simulink model "exm070102"  (R2018a)
settings: Solver=ode45  StartTime=0.0  StopTime=10  MaxStep=0.01  RelTol=1e-3  EnableMultiTasking=on
settings Model: Creator=acer  LastModifiedBy=zyzhang
settings DataIOCC: LimitDataPoints=on  SaveFormat=Array  SignalLoggingSaveFormat=ModelDataLogs
settings OptimizationCC: ExpressionDepthLimit=2147483647  LifeSpan=inf
settings DebuggingCC: UnderspecifiedInitializationDetection=Classic  MergeDetectMultiDrivingBlocksExec=none  SolverPrmCheckMsg=warning  FcnCallInpInsideContextMsg=warning  StateNameClashWarn=warning  SFUnexpectedBacktrackingDiag=warning  SFNoUnconditionalDefaultTransitionDiag=warning  SFExecutionAtInitializationDiag=none
settings HardwareCC: ProdBitPerPointer=32  ProdBitPerSizeT=32  ProdBitPerPtrDiffT=32  ProdLargestAtomicFloat=None  ProdIntDivRoundTo=Undefined  ProdEndianess=Unspecified  ProdWordSize=32  ProdHWDeviceType=32-bit Generic
settings ModelReferenceCC: PropagateSignalLabelsOutOfModel=off
settings CodeAppCC: StateflowObjectComments=on
settings GRTTargetCC: TargetLangStandard=C89/C90 (ANSI)  GeneratePreprocessorConditionals=Disable all  CombineOutputUpdateFcns=off  GRTInterface=on
settings ConfigComp: CovMetricSettings=dw  CovHtmlReporting=on  CovSaveCumulativeToWorkspaceVar=on  CovSaveSingleToWorkspaceVar=on  CovExternalEMLEnable=off  CovSFcnEnable=off

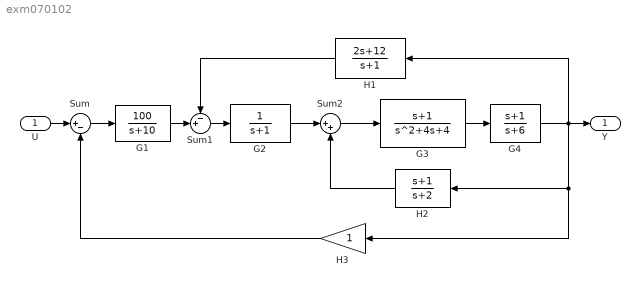
== system exm070102 ==
  U : Inport
  G1 : TransferFcn  Numerator=[100]  Denominator=[1 10]
  G2 : TransferFcn  Denominator=[1 1]
  G3 : TransferFcn  Numerator=[1 1]  Denominator=[1 4 4]
  G4 : TransferFcn  Numerator=[1 1]  Denominator=[1 6]
  H1 : TransferFcn  Numerator=[2 12]  Denominator=[1 1]
  H2 : TransferFcn  Numerator=[1 1]  Denominator=[1 2]
  H3 : Gain
  Sum : Sum  Inputs=|+-
  Sum1 : Sum  Inputs=-+|
  Sum2 : Sum  Inputs=|++
  Y : Outport
  wires:
  U/1 -> Sum/1
  Sum/1 -> G1/1
  Sum1/1 -> G2/1
  G2/1 -> Sum2/1
  Sum2/1 -> G3/1
  G3/1 -> G4/1
  G4/1 -> H1/1, H2/1, H3/1, Y/1
  G1/1 -> Sum1/2
  H1/1 -> Sum1/1
  H2/1 -> Sum2/2
  H3/1 -> Sum/2
